simulink model "model2LAB1"  (R2020a)
settings: Solver=VariableStepAuto  StartTime=0.0  StopTime=127  RelTol=1e-3
libraries: simulink_extras x1, commrandsrc3 x1
settings Model: Creator=Sameer  LastModifiedBy=Sameer

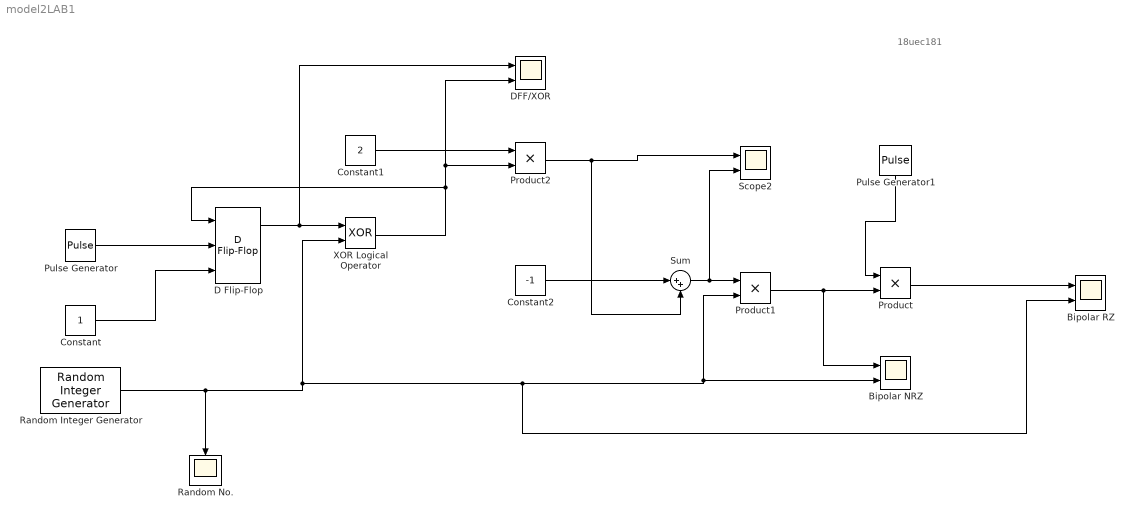
== system model2LAB1 ==
  note: 18uec181
  Bipolar NRZ : Scope  NumInputPorts=2
  Bipolar RZ : Scope  NumInputPorts=2
  Constant : Constant
  Constant1 : Constant  Value=2
  Constant2 : Constant  Value=-1
  D Flip-Flop : simulink_extras/Flip Flops/D Flip-Flop
  DFF/XOR : Scope  NumInputPorts=2
  Product : Product
  Product1 : Product
  Product2 : Product
  Pulse Generator : DiscretePulseGenerator  PulseType=Time based  Period=1  PulseWidth=50
  Pulse Generator1 : DiscretePulseGenerator  PulseType=Time based  Period=1  PulseWidth=50
  Random Integer Generator : commrandsrc3/Random Integer Generator  SetSize=2  SeedSource=Auto  Seed=0  SampleTime=1  SamplesPerFrame=1  OutputDataType=double  SimulateUsing=Interpreted execution
  Random No. : Scope
  Scope2 : Scope  NumInputPorts=2
  Sum : Sum  Inputs=|++
  XOR Logical Operator : Logic  Operator=XOR  AllPortsSameDT=off  OutDataTypeStr=boolean
  wires:
  Constant/1 -> D Flip-Flop/3
  Pulse Generator/1 -> D Flip-Flop/2
  D Flip-Flop/1 -> XOR Logical Operator/1, DFF/XOR/1
  Constant1/1 -> Product2/1
  Product2/1 -> Sum/2, Scope2/1
  Random Integer Generator/1 -> Bipolar RZ/2, Bipolar NRZ/2, Product1/2, XOR Logical Operator/2, Random No./1
  XOR Logical Operator/1 -> D Flip-Flop/1, Product2/2, DFF/XOR/2
  Constant2/1 -> Sum/1
  Sum/1 -> Scope2/2, Product1/1
  Pulse Generator1/1 -> Product/1
  Product1/1 -> Bipolar NRZ/1, Product/2
  Product/1 -> Bipolar RZ/1
